simulink model "bangcontrol"  (R2021b)
settings: Solver=ode3  StartTime=0.0  StopTime=300  FixedStep=0.5  RelTol=1e-3  EnableMultiTasking=on
libraries: arduinolib x2
settings Model: ExtModeTrigDuration=2  Creator=tsuga  LastModifiedBy=karteek
settings DataIOCC: SaveOutput=off  SignalLogging=off  DSMLogging=off  SaveTime=off  ReturnWorkspaceOutputs=off
settings OptimizationCC: EnhancedBackFolding=on  PassReuseOutputArgsAs=Individual arguments  ZeroExternalMemoryAtStartup=off  ZeroInternalMemoryAtStartup=off  MaxStackSize=64  OptimizeBlockOrder=speed  DifferentSizesBufferReuse=on  OptimizationCustomize=off  EfficientTunableParamExpr=on
settings DebuggingCC: ParameterTunabilityLossMsg=error
settings HardwareCC: ProdBitPerInt=16  ProdBitPerPointer=16  ProdBitPerSizeT=16  ProdBitPerPtrDiffT=16  ProdLargestAtomicFloat=None  ProdWordSize=8  ProdHWDeviceType=Atmel->AVR
settings SFSimCC: MATLABDynamicMemAlloc=off
settings RTWCC: Description=Embedded Coder  SystemTargetFile=ert.tlc  HardwareBoard=Arduino Leonardo  TemplateMakefile=ert_default_tmf  Toolchain=Arduino AVR  BuildConfiguration=Faster Runs
settings CodeAppCC: ForceParamTrailComments=on  IgnoreCustomStorageClasses=off  OperatorAnnotations=on  SimulinkDataObjDesc=on  SFDataObjDesc=on  InsertBlockDesc=on
settings ERTTargetCC: SupportContinuousTime=on  SupportVariableSizeSignals=on  ExtModeTransport=5  ExtModeStaticAllocSize=250  ExtModeMexFile=ext_serial_win32_comm_leonardo

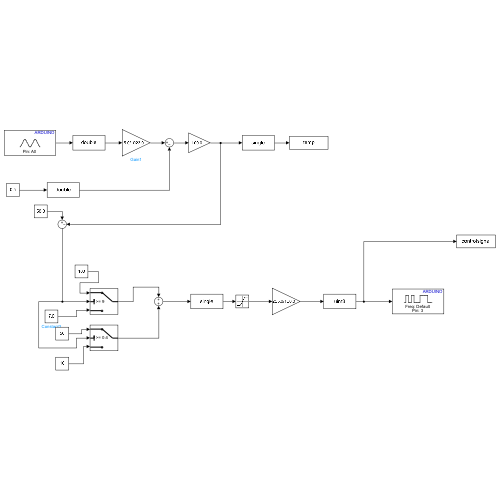
[thumbnail: Simulink's stored preview of the top-level diagram]
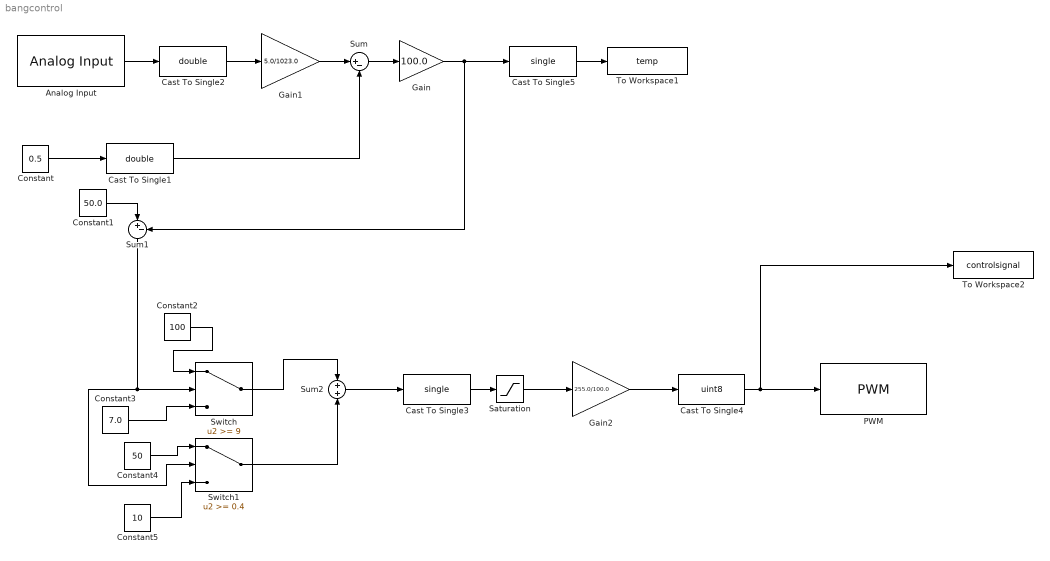
== system bangcontrol ==
  Analog Input : arduinolib/Analog Input  pinNumber=0  ReadResultsOnly=off  ConversionTriggerSource=Software  ExternalTriggerType=uint32( 0 )  OutputDataType=uint16  EnableConversionCompleteNotify=off  EnableOuputStatus=off  SampleTime=0.5  blockPlatform=arduino
  Cast To Single1 : DataTypeConversion  OutDataTypeStr=double
  Cast To Single2 : DataTypeConversion  OutDataTypeStr=double
  Cast To Single3 : DataTypeConversion  OutDataTypeStr=single
  Cast To Single4 : DataTypeConversion  OutDataTypeStr=uint8
  Cast To Single5 : DataTypeConversion  OutDataTypeStr=single
  Constant : Constant  Value=0.5  SampleTime=0.5
  Constant1 : Constant  Value=50.0  SampleTime=0.5
  Constant2 : Constant  Value=100  SampleTime=0.5
  Constant3 : Constant  Value=7.0  SampleTime=0.5
  Constant4 : Constant  Value=50  SampleTime=0.5
  Constant5 : Constant  Value=10  SampleTime=0.5
  Gain : Gain  Gain=100.0
  Gain1 : Gain  Gain=5.0/1023.0
  Gain2 : Gain  Gain=255.0/100.0
  PWM : arduinolib/PWM  pinNumber=3  frequencyType=Default  desiredFrequency=490.2  achievableFrequency=490.2
  Saturation : Saturate  UpperLimit=100.0  LowerLimit=0.0
  Sum : Sum  Inputs=|+-
  Sum1 : Sum  Inputs=|+-
  Sum2 : Sum
  Switch : Switch  Threshold=9
  Switch1 : Switch  Threshold=0.4
  To Workspace1 : ToWorkspace  VariableName=temp  SampleTime=0.5
      settings: Save2DSignal=2-D array (concatenate along first dimension)
  To Workspace2 : ToWorkspace  VariableName=controlsignal  SampleTime=0.5
      settings: Save2DSignal=2-D array (concatenate along first dimension)
  wires:
  Constant/1 -> Cast To Single1/1
  Sum/1 -> Gain/1
  Gain/1 -> Sum1/2, Cast To Single5/1
  Cast To Single1/1 -> Sum/2
  Gain1/1 -> Sum/1
  Analog Input/1 -> Cast To Single2/1
  Cast To Single2/1 -> Gain1/1
  Cast To Single3/1 -> Saturation/1
  Saturation/1 -> Gain2/1
  Gain2/1 -> Cast To Single4/1
  Cast To Single4/1 -> To Workspace2/1, PWM/1
  Cast To Single5/1 -> To Workspace1/1
  Constant1/1 -> Sum1/1
  Sum1/1 -> Switch1/2, Switch/2
  Constant2/1 -> Switch/1
  Constant3/1 -> Switch/3
  Constant4/1 -> Switch1/1
  Switch1/1 -> Sum2/2
  Switch/1 -> Sum2/1
  Sum2/1 -> Cast To Single3/1
  Constant5/1 -> Switch1/3
